simulink model "Simulacao_PID"  (R2015a)
settings: Solver=ode45  StartTime=0.0  StopTime=1000  RelTol=1e-3
libraries: simulink x1
settings Model: Creator=gabri  LastModifiedBy=gabri
settings DataIOCC: LimitDataPoints=off

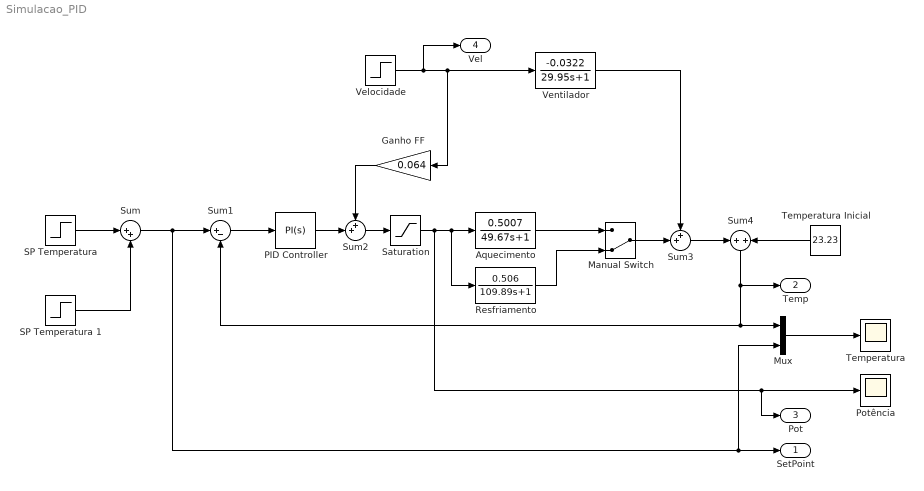
== system Simulacao_PID ==
  Aquecimento : TransferFcn  Numerator=[0.5007]  Denominator=[49.67 1]
  Ganho FF : Gain  Gain=0.064
  Manual Switch : ManualSwitch  CurrentSetting=0
  Mux : Mux  Inputs=2
  PID Controller : simulink/Continuous/PID Controller  Controller=PI  TimeDomain=Continuous-time  SampleTime=-1  IntegratorMethod=Forward Euler  FilterMethod=Forward Euler  Form=Parallel  UseFilter=on  ControllerParametersSource=internal  P=3  I=0.07  D=0  N=100  InitialConditionSource=internal  InitialConditionForIntegrator=0  InitialConditionForFilter=0  ExternalReset=none  LimitOutput=on  UpperSaturationLimit=100  LowerSaturationLimit=0  LinearizeAsGain=on  AntiWindupMode=back-calculation  Kb=1  TrackingMode=off  Kt=1  PParamMin=[]  PParamMax=[]  IParamMin=[]  IParamMax=[]  DParamMin=[]  DParamMax=[]  NParamMin=[]  NParamMax=[]  KbParamMin=[]  KbParamMax=[]  KtParamMin=[]  KtParamMax=[]  POutMin=[]  POutMax=[]  IOutMin=[]  IOutMax=[]  DOutMin=[]  DOutMax=[]  NOutMin=[]  NOutMax=[]  KbOutMin=[]  KbOutMax=[]  KtOutMin=[]  KtOutMax=[]  IntegratorOutMin=[]  IntegratorOutMax=[]  FilterOutMin=[]  FilterOutMax=[]  SumOutMin=[]  SumOutMax=[]  SumI1OutMin=[]  SumI1OutMax=[]  SumI2OutMin=[]  SumI2OutMax=[]  SumI3OutMin=[]  SumI3OutMax=[]  SumDOutMin=[]  SumDOutMax=[]  SaturationOutMin=[]  SaturationOutMax=[]  IntegratorContinuousStateAttributes=''  IntegratorStateMustResolveToSignalObject=off  IntegratorRTWStateStorageClass=Auto  FilterContinuousStateAttributes=''  FilterStateMustResolveToSignalObject=off  FilterRTWStateStorageClass=Auto  DifferentiatorICPrevScaledInput=0  DifferentiatorOutMin=[]  DifferentiatorOutMax=[]
  Potência : Scope
  Resfriamento : TransferFcn  Numerator=[0.506]  Denominator=[109.89 1]
  "SP Temperatura " : Step  Time=10  Before=23.3  After=55  SampleTime=1
  SP Temperatura 1 : Step  Time=600  After=-15  SampleTime=1
  Saturation : Saturate  UpperLimit=100  LowerLimit=0
  Sum : Sum  Inputs=|++
  Sum1 : Sum  Inputs=|+-
  Sum2 : Sum  Inputs=++|
  Sum3 : Sum  Inputs=++|
  Sum4 : Sum  Inputs=+|+
  Temperatura : Scope
  Temperatura Inicial : Constant  Value=23.23
  Velocidade : Step  Time=0  After=0  SampleTime=1
  "Ventilador " : TransferFcn  Numerator=[-0.0322]  Denominator=[29.95 1]
  SetPoint : Outport
  Temp : Outport  Port=2
  Pot : Outport  Port=3
  Vel : Outport  Port=4
  wires:
  "SP Temperatura "/1 -> Sum/1
  Sum/1 -> SetPoint/1, Mux/2, Sum1/1
  Sum1/1 -> PID Controller/1
  PID Controller/1 -> Sum2/2
  Manual Switch/1 -> Sum3/2
  Velocidade/1 -> Vel/1, Ganho FF/1, "Ventilador "/1
  Sum3/1 -> Sum4/1
  Mux/1 -> Temperatura/1
  Sum4/1 -> Temp/1, Sum1/2, Mux/1
  Temperatura Inicial/1 -> Sum4/2
  Aquecimento/1 -> Manual Switch/1
  Resfriamento/1 -> Manual Switch/2
  "Ventilador "/1 -> Sum3/1
  SP Temperatura 1/1 -> Sum/2
  Ganho FF/1 -> Sum2/1
  Saturation/1 -> Aquecimento/1, Resfriamento/1, Pot/1, Potência/1
  Sum2/1 -> Saturation/1
